simulink model "tx80211a2l"  (R2015b)
settings: Solver=FixedStepDiscrete  SolverMode=SingleTasking  StartTime=0.0  StopTime=46*tpf  RelTol=1e-3
PreLoadFcn:
  | [stx, stb, spi, spq, ntf, cii, cpp, css] = tx80211a_r0;
InitFcn:
  | if ~exist('srx','var')
  | [stx, stb, spi, spq, ntf, cii, cpp, css] = tx80211a_r0;
  | end
  | bitrate = 6e6; % 6 Mbits per second
  | crf = 2; % constant redundancy factor (from conv enc)
  | nepsc = 16; % #empty+pilot subcarriers
  | ncps = 16; % #cyclic prefix samples
  | ndbpf = 24; % #data bits per frame
  | ncbpf = ndbpf * crf; % #coded bits per frame
  | nscpf = ncbpf + nepsc; % #subcarriers per frame
  | nspf = nscpf + 16; % #samples per frame
  | tps = 1e-6; %tpf/nspf; % sample time
  | tpf = tps*nspf; %ndbpf/bitrate; % frame time
undefined symbols (not defined in the file): cpp, css, ntf, Radix, spi, spq, stb
libraries: hdlsllib x30, simulink x20, commdigbbndpm3 x1, commcnvcod2 x1, dspxfrm3 x1
settings Model: Creator=wchen  LastModifiedBy=bdroz
settings SolverCC: PositivePriorityOrder=on
settings DataIOCC: SaveFormat=Array  SaveOutput=off  SignalLogging=off  SaveTime=off
settings OptimizationCC: BlockReduction=off  ConditionallyExecuteInputs=off  DefaultParameterBehavior=Inlined  ExpressionDepthLimit=2147483647  OptimizeModelRefInitCode=on  LifeSpan=1  MaxStackSize=64
settings DebuggingCC: AlgebraicLoopMsg=error  UnderspecifiedInitializationDetection=Classic  MergeDetectMultiDrivingBlocksExec=none  SolverPrmCheckMsg=warning  SingleTaskRateTransMsg=error  ParameterPrecisionLossMsg=none  AllowSymbolicDim=on  StateNameClashWarn=warning
settings HardwareCC: ProdBitPerPointer=32  ProdLargestAtomicFloat=None  ProdIntDivRoundTo=Undefined  ProdEndianess=Unspecified  ProdWordSize=32  ProdHWDeviceType=ASIC/FPGA->ASIC/FPGA  TargetBitPerPointer=64  TargetLongLongMode=on  TargetIntDivRoundTo=Zero  TargetEndianess=LittleEndian  TargetWordSize=64  TargetHWDeviceType=MATLAB Host  ProdEqTarget=off
settings RTWCC: SystemTargetFile=ert.tlc  TemplateMakefile=ert_default_tmf  Description=Embedded Coder  GenerateReport=on  Toolchain=Xilinx Software Development Kit (SDK)  IncludeHyperlinkInReport=on  LaunchReport=on  GenerateTraceInfo=on  GenerateTraceReport=on  GenerateTraceReportSl=on  GenerateTraceReportSf=on  GenerateTraceReportEml=on
settings CodeAppCC: ForceParamTrailComments=on  IgnoreCustomStorageClasses=off  OperatorAnnotations=on  SimulinkDataObjDesc=on  SFDataObjDesc=on  MATLABFcnDesc=on  InsertBlockDesc=on  MATLABSourceComments=on
settings ERTTargetCC: ERTCustomFileTemplate=example_file_process.tlc  ConvertIfToSwitch=on  SuppressUnreachableDefaultCases=on
settings ConfigComp: CovModelRefEnable=Off

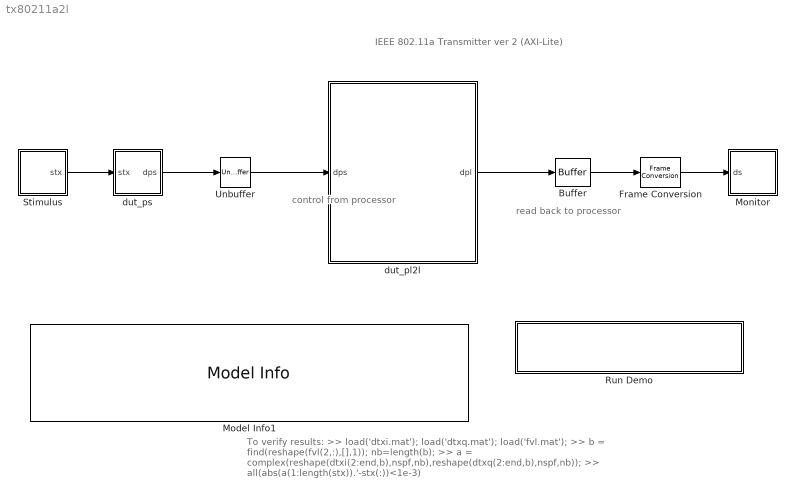
== system tx80211a2l ==
  note: control from
      | processor
  note: IEEE 802.11a Transmitter ver 2 (AXI-Lite)
  note: read back to
      | processor
  note: To verify results:
      | >> load('dtxi.mat'); load('dtxq.mat'); load('fvl.mat');
      | >> b = find(reshape(fvl(2,:),[],1)); nb=length(b);
      | >> a = complex(reshape(dtxi(2:end,b),nspf,nb),reshape(dtxq(2:end,b),nspf,nb));
      | >> all(abs(a(1:length(stx)).'-stx(:))<1e-3)
  Buffer : Buffer  N=80  TreatMby1Signals=One channel  OutputFrames=off
  Frame Conversion : FrameConversion  InheritSamplingMode=off  OutFrame=Sample-based
  Model Info1 : simulink/Model-Wide Utilities/Model Info  Frame=on  DisplayStringWithTags=|  HorizontalTextAlignment=Left  LeftAlignmentValue=0.02  SourceBlockDiagram=tx80211a2l  TagMaxNumber=20
      | This example shows how to use HDL Workflow Advisor to 
      | generate a custom IP core for Zynq SoC evaluation board.
      | 
      | In MATLAB, type the following:
      |   hdladvisor('tx80211a2l/dut_pl2l')
  Monitor : Subsystem
  Run Demo : Subsystem
      settings: OpenFcn=hdladvisor([bdroot, '/led_counter'])
      mask Display: disp('Launch HDL Workflow Advisor')
  Stimulus : Subsystem
  Unbuffer : Unbuffer  SampleBasedProcessing=Same as frame based
  dut_pl2l : Subsystem  TreatAsAtomicUnit=on
  dut_ps : Subsystem
  wires:
  Buffer/1 -> Frame Conversion/1
  dut_pl2l/1(dpl) -> Buffer/1
  Stimulus/1(stx) -> dut_ps/1(stx)
  dut_ps/1(dps) -> Unbuffer/1
  Unbuffer/1 -> dut_pl2l/1(dps)
  Frame Conversion/1 -> Monitor/1(ds)

== system tx80211a2l/Monitor ==
  ds : Inport
  Compare To Constant : simulink/Logic and Bit Operations/Compare To Constant  relop=>  const=uint16(0)  OutDataTypeStr=boolean
  Counter Free-Running : simulink/Sources/Counter Free-Running  NumBits=16  tsamp=tpf
  Unpack_int32_into_fix16c1b : Subsystem
  write_srb_to_file : Subsystem
  wires:
  Compare To Constant/1 -> write_srb_to_file/Enable
  Counter Free-Running/1 -> Compare To Constant/1
  ds/1 -> Unpack_int32_into_fix16c1b/1(di32)
  Unpack_int32_into_fix16c1b/2(fvd) -> write_srb_to_file/2(fvl)
  Unpack_int32_into_fix16c1b/1(dts) -> write_srb_to_file/1(srb)

== system tx80211a2l/Run Demo ==

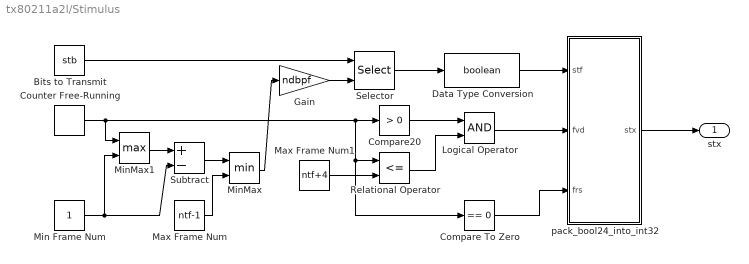
== system tx80211a2l/Stimulus ==
  Bits to Transmit : Constant  Value=stb  SampleTime=tpf
  Compare To Zero : simulink/Logic and Bit Operations/Compare To Zero  relop===  OutDataTypeStr=boolean
  Compare20 : simulink/Logic and Bit Operations/Compare To Zero  relop=>  OutDataTypeStr=boolean
  Counter Free-Running : simulink/Sources/Counter Free-Running  NumBits=16  tsamp=tpf
  Data Type Conversion : DataTypeConversion  OutDataTypeStr=boolean
  Gain : Gain  Gain=ndbpf  OutDataTypeStr=uint16
  Logical Operator : Logic  AllPortsSameDT=off  OutDataTypeStr=boolean
  Max Frame Num : Constant  Value=ntf-1  OutDataTypeStr=uint16  SampleTime=tpf
  Max Frame Num1 : Constant  Value=ntf+4  OutDataTypeStr=uint16  SampleTime=tpf
  Min Frame Num : Constant  OutDataTypeStr=uint16  SampleTime=tpf
  MinMax : MinMax  Inputs=2  OutDataTypeStr=uint16
  MinMax1 : MinMax  Function=max  Inputs=2
  Relational Operator : RelationalOperator  Operator=<=  OutDataTypeStr=boolean
  Selector : Selector  IndexMode=Zero-based  InputPortWidth=864  IndexOptions=Starting index (port)  Indices=[1 3]  OutputSizes=24
  Subtract : Sum  Inputs=+-  OutDataTypeStr=uint16
  pack_bool24_into_int32 : Subsystem
  stx : Outport
  wires:
  Compare To Zero/1 -> pack_bool24_into_int32/3(frs)
  MinMax1/1 -> Subtract/1
  Subtract/1 -> MinMax/1
  Min Frame Num/1 -> MinMax1/2, Subtract/2
  pack_bool24_into_int32/1(stx) -> stx/1
  Data Type Conversion/1 -> pack_bool24_into_int32/1(stf)
  Selector/1 -> Data Type Conversion/1
  Gain/1 -> Selector/2
  Bits to Transmit/1 -> Selector/1
  MinMax/1 -> Gain/1
  Max Frame Num/1 -> MinMax/2
  Counter Free-Running/1 -> Compare20/1, Relational Operator/1, Compare To Zero/1, MinMax1/1
  Compare20/1 -> Logical Operator/1
  Relational Operator/1 -> Logical Operator/2
  Logical Operator/1 -> pack_bool24_into_int32/2(fvd)
  Max Frame Num1/1 -> Relational Operator/2

== system tx80211a2l/dut_pl2l ==
  dps : Inport
  Preamble Switch : Subsystem  TreatAsAtomicUnit=on
  Unpack_int32_into_fix16c2b : Subsystem
  pack_fpt16c1b_into_int32 : Subsystem
  dpl : Outport
  wires:
  dps/1 -> Unpack_int32_into_fix16c2b/1(di32)
  Unpack_int32_into_fix16c2b/1(dts) -> Preamble Switch/1(s8s)
  Unpack_int32_into_fix16c2b/2(fvd) -> Preamble Switch/2(f8v)
  Preamble Switch/1(s9s) -> pack_fpt16c1b_into_int32/1(dtf16c)
  pack_fpt16c1b_into_int32/1(dti32) -> dpl/1
  Preamble Switch/2(f9v) -> pack_fpt16c1b_into_int32/2(fvd)
  Unpack_int32_into_fix16c2b/3(frs) -> Preamble Switch/3(frs)

== system tx80211a2l/dut_ps ==
  stx : Inport
  Logical AND : Logic  IconShape=distinctive  AllPortsSameDT=off  OutDataTypeStr=boolean
  pack_fpt16c_into_int32 : Subsystem
  prepare_frame_ps : Subsystem  TreatAsAtomicUnit=on
  unpack_int32_into_bool24 : Subsystem
  dps : Outport
  wires:
  stx/1 -> unpack_int32_into_bool24/1(di32)
  unpack_int32_into_bool24/3(frs) -> pack_fpt16c_into_int32/3(frs), prepare_frame_ps/2(frs)
  unpack_int32_into_bool24/1(stx) -> prepare_frame_ps/1(stb)
  unpack_int32_into_bool24/2(fvd) -> Logical AND/2, prepare_frame_ps/Enable
  prepare_frame_ps/2(fvo) -> Logical AND/1
  prepare_frame_ps/1(dts) -> pack_fpt16c_into_int32/1(dtf16c)
  Logical AND/1 -> pack_fpt16c_into_int32/2(fvd)
  pack_fpt16c_into_int32/1(dti32) -> dps/1

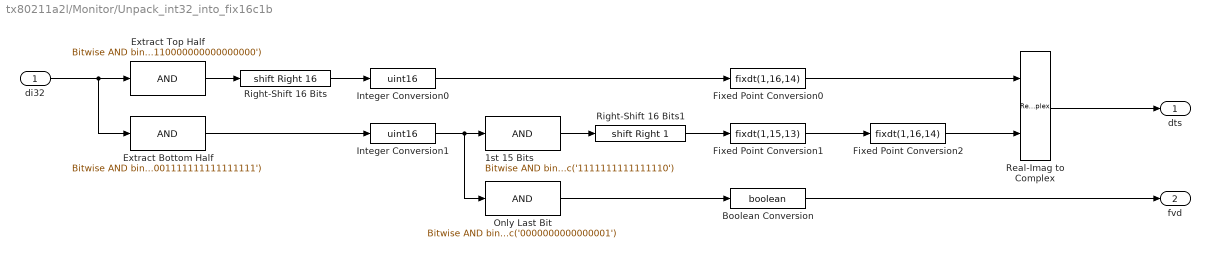
== system tx80211a2l/Monitor/Unpack_int32_into_fix16c1b ==
  di32 : Inport
  1st 15 Bits : simulink/Logic and Bit Operations/Bitwise Operator  logicop=AND  UseBitMask=on  BitMask=bin2dec('1111111111111110')  BitMaskRealWorld=Stored Integer
  Boolean Conversion : DataTypeConversion  OutDataTypeStr=boolean  ConvertRealWorld=Stored Integer (SI)
  Extract Bottom Half : simulink/Logic and Bit Operations/Bitwise Operator  logicop=AND  UseBitMask=on  BitMask=bin2dec('00000000000000001111111111111111')  BitMaskRealWorld=Stored Integer
  Extract Top Half : simulink/Logic and Bit Operations/Bitwise Operator  logicop=AND  UseBitMask=on  BitMask=bin2dec('11111111111111110000000000000000')  BitMaskRealWorld=Stored Integer
  Fixed Point Conversion0 : DataTypeConversion  OutDataTypeStr=fixdt(1,16,14)  ConvertRealWorld=Stored Integer (SI)
      settings: AttributesFormatString=%<OutDataTypeStr>
  Fixed Point Conversion1 : DataTypeConversion  OutDataTypeStr=fixdt(1,15,13)  ConvertRealWorld=Stored Integer (SI)
      settings: AttributesFormatString=%<OutDataTypeStr>
  Fixed Point Conversion2 : DataTypeConversion  OutDataTypeStr=fixdt(1,16,14)
      settings: AttributesFormatString=%<OutDataTypeStr>
  Integer Conversion0 : DataTypeConversion  OutDataTypeStr=uint16  ConvertRealWorld=Stored Integer (SI)
  Integer Conversion1 : DataTypeConversion  OutDataTypeStr=uint16  ConvertRealWorld=Stored Integer (SI)
  Only Last Bit : simulink/Logic and Bit Operations/Bitwise Operator  logicop=AND  UseBitMask=on  BitMask=bin2dec('0000000000000001')  BitMaskRealWorld=Stored Integer
  Real-Imag to Complex : RealImagToComplex
  Right-Shift 16 Bits : ArithShift  BitShiftNumber=16  BitShiftDirection=Right  DiagnosticForOORShift=Error
  Right-Shift 16 Bits1 : ArithShift  BitShiftNumber=1  BitShiftDirection=Right  DiagnosticForOORShift=Error
  dts : Outport
  fvd : Outport  Port=2
  wires:
  Real-Imag to Complex/1 -> dts/1
  Only Last Bit/1 -> Boolean Conversion/1
  Boolean Conversion/1 -> fvd/1
  Fixed Point Conversion0/1 -> Real-Imag to Complex/1
  Fixed Point Conversion2/1 -> Real-Imag to Complex/2
  Extract Bottom Half/1 -> Integer Conversion1/1
  di32/1 -> Extract Bottom Half/1, Extract Top Half/1
  1st 15 Bits/1 -> Right-Shift 16 Bits1/1
  Right-Shift 16 Bits/1 -> Integer Conversion0/1
  Extract Top Half/1 -> Right-Shift 16 Bits/1
  Integer Conversion1/1 -> 1st 15 Bits/1, Only Last Bit/1
  Integer Conversion0/1 -> Fixed Point Conversion0/1
  Fixed Point Conversion1/1 -> Fixed Point Conversion2/1
  Right-Shift 16 Bits1/1 -> Fixed Point Conversion1/1

== system tx80211a2l/Monitor/write_srb_to_file ==
  srb : Inport
  fvl : Inport  Port=2
  Enable : EnablePort
  Complex to Real-Imag : ComplexToRealImag
  Data Type Conversion : DataTypeConversion  OutDataTypeStr=double
  Data Type Conversion1 : DataTypeConversion  OutDataTypeStr=double
  To File : ToFile  Filename=dtxi.mat  MatrixName=dtxi  SampleTime=tpf
  To File1 : ToFile  Filename=fvl.mat  MatrixName=fvl  SampleTime=tpf
  To File2 : ToFile  Filename=dtxq.mat  MatrixName=dtxq  SampleTime=tpf
  wires:
  fvl/1 -> Data Type Conversion1/1
  Data Type Conversion1/1 -> To File1/1
  srb/1 -> Data Type Conversion/1
  Data Type Conversion/1 -> Complex to Real-Imag/1
  Complex to Real-Imag/1 -> To File/1
  Complex to Real-Imag/2 -> To File2/1

== system tx80211a2l/Stimulus/pack_bool24_into_int32 ==
  stf : Inport
  fvd : Inport  Port=2
  frs : Inport  Port=3
  Bit Concat : hdlsllib/HDL Operations/Bit Concat  numInputs=1
  Constant : Constant  Value=false(6,1)  OutDataTypeStr=boolean  SampleTime=tpf
  Vector Concatenate : Concatenate  NumInputs=4
  stx : Outport
  wires:
  Vector Concatenate/1 -> Bit Concat/1
  stf/1 -> Vector Concatenate/1
  fvd/1 -> Vector Concatenate/3
  frs/1 -> Vector Concatenate/4
  Constant/1 -> Vector Concatenate/2
  Bit Concat/1 -> stx/1

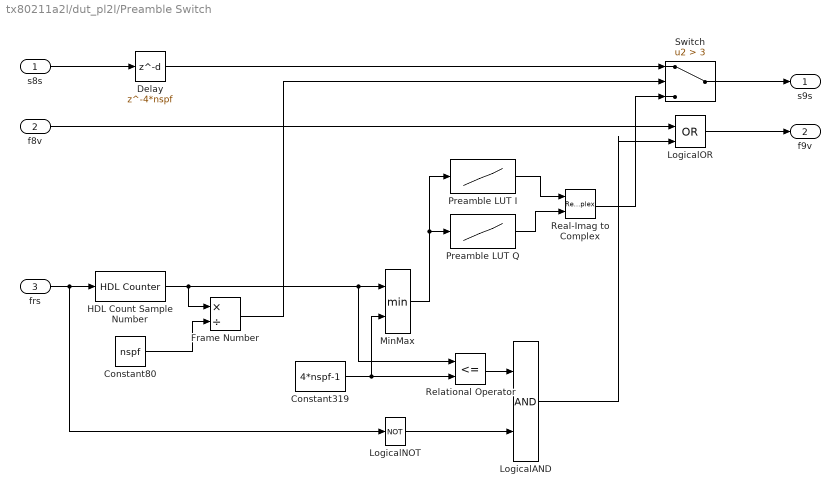
== system tx80211a2l/dut_pl2l/Preamble Switch ==
  s8s : Inport
  f8v : Inport  Port=2
  frs : Inport  Port=3
  Constant319 : Constant  Value=4*nspf-1  OutDataTypeStr=uint16  SampleTime=tps
  Constant80 : Constant  Value=nspf  OutDataTypeStr=uint8  SampleTime=tps
  Delay : Delay  DelayLength=4*nspf  SampleTime=tps
  Frame Number : Product  Inputs=*/  OutDataTypeStr=uint16  SaturateOnIntegerOverflow=on  RndMeth=Zero
  HDL Count Sample Number : hdlsllib/HDL Operations/HDL Counter  CountType=Free running  CountInit=0  CountStep=1  CountMax=3  CountFromType=Initial value  CountFrom=0  CountResetPort=on  CountLoadPort=off  CountEnbPort=off  CountDirPort=off  CountDataType=Unsigned  CountWordLen=16  CountFracLen=0  CountSampTime=1
  LogicalAND : Logic  IconShape=distinctive  AllPortsSameDT=off  OutDataTypeStr=boolean
  LogicalNOT : Logic  Operator=NOT  IconShape=distinctive  AllPortsSameDT=off  OutDataTypeStr=boolean
  LogicalOR : Logic  Operator=OR  IconShape=distinctive  AllPortsSameDT=off  OutDataTypeStr=boolean
  MinMax : MinMax  Inputs=2
  Preamble LUT I : Lookup_n-D  NumberOfTableDimensions=1  BreakpointsForDimension1=[0:1:319]  BreakpointsForDimension1FirstPoint=10  BreakpointsForDimension2FirstPoint=10  BreakpointsForDimension1Spacing=12  BreakpointsForDimension2Spacing=12  IndexSearchMethod=Evenly spaced points  Table=spi  InterpMethod=Flat  DiagnosticForOutOfRangeInput=Error  InternalRulePriority=Speed  OutDataTypeStr=fixdt(1,16,14)  RndMeth=Simplest  InputSameDT=on
  Preamble LUT Q : Lookup_n-D  NumberOfTableDimensions=1  BreakpointsForDimension1=[0:1:319]  BreakpointsForDimension1FirstPoint=10  BreakpointsForDimension2FirstPoint=10  BreakpointsForDimension1Spacing=12  BreakpointsForDimension2Spacing=12  IndexSearchMethod=Evenly spaced points  Table=spq  TableDataTypeStr=fixdt(1,16,14)  InterpMethod=Flat  DiagnosticForOutOfRangeInput=Error  InternalRulePriority=Speed  OutDataTypeStr=fixdt(1,16,14)  RndMeth=Simplest  InputSameDT=on
  Real-Imag to Complex : RealImagToComplex
  Relational Operator : RelationalOperator  Operator=<=  OutDataTypeStr=boolean
  Switch : Switch  Criteria=u2 > Threshold  Threshold=3
  s9s : Outport
  f9v : Outport  Port=2
  wires:
  frs/1 -> LogicalNOT/1, HDL Count Sample Number/1
  Switch/1 -> s9s/1
  s8s/1 -> Delay/1
  Real-Imag to Complex/1 -> Switch/3
  Constant80/1 -> Frame Number/2
  Delay/1 -> Switch/1
  Frame Number/1 -> Switch/2
  HDL Count Sample Number/1 -> Relational Operator/1, MinMax/1, Frame Number/1
  Constant319/1 -> MinMax/2, Relational Operator/2
  MinMax/1 -> Preamble LUT Q/1, Preamble LUT I/1
  LogicalOR/1 -> f9v/1
  LogicalNOT/1 -> LogicalAND/2
  Relational Operator/1 -> LogicalAND/1
  LogicalAND/1 -> LogicalOR/2
  f8v/1 -> LogicalOR/1
  Preamble LUT I/1 -> Real-Imag to Complex/1
  Preamble LUT Q/1 -> Real-Imag to Complex/2

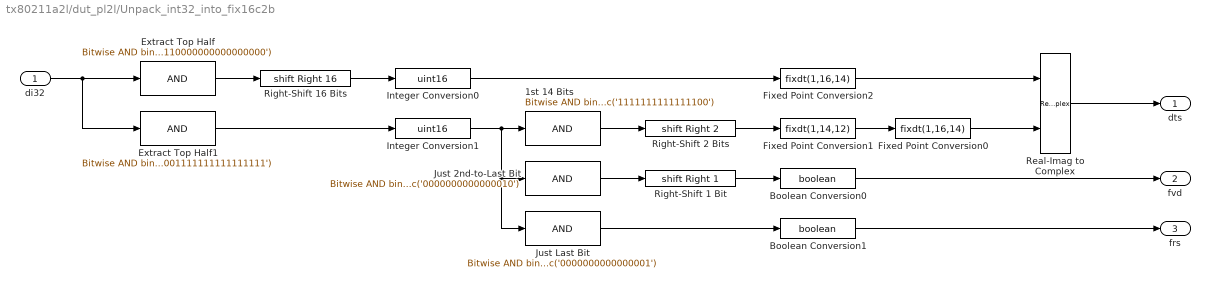
== system tx80211a2l/dut_pl2l/Unpack_int32_into_fix16c2b ==
  di32 : Inport
  1st 14 Bits : simulink/Logic and Bit Operations/Bitwise Operator  logicop=AND  UseBitMask=on  BitMask=bin2dec('1111111111111100')  BitMaskRealWorld=Stored Integer
  Boolean Conversion0 : DataTypeConversion  OutDataTypeStr=boolean  ConvertRealWorld=Stored Integer (SI)
  Boolean Conversion1 : DataTypeConversion  OutDataTypeStr=boolean  ConvertRealWorld=Stored Integer (SI)
  Extract Top Half : simulink/Logic and Bit Operations/Bitwise Operator  logicop=AND  UseBitMask=on  BitMask=bin2dec('11111111111111110000000000000000')  BitMaskRealWorld=Stored Integer
  Extract Top Half1 : simulink/Logic and Bit Operations/Bitwise Operator  logicop=AND  UseBitMask=on  BitMask=bin2dec('00000000000000001111111111111111')  BitMaskRealWorld=Stored Integer
  Fixed Point Conversion0 : DataTypeConversion  OutDataTypeStr=fixdt(1,16,14)  LockScale=on
      settings: AttributesFormatString=%<OutDataTypeStr>
  Fixed Point Conversion1 : DataTypeConversion  OutDataTypeStr=fixdt(1,14,12)  ConvertRealWorld=Stored Integer (SI)  LockScale=on
      settings: AttributesFormatString=%<OutDataTypeStr>
  Fixed Point Conversion2 : DataTypeConversion  OutDataTypeStr=fixdt(1,16,14)  ConvertRealWorld=Stored Integer (SI)
      settings: AttributesFormatString=%<OutDataTypeStr>
  Integer Conversion0 : DataTypeConversion  OutDataTypeStr=uint16  ConvertRealWorld=Stored Integer (SI)
  Integer Conversion1 : DataTypeConversion  OutDataTypeStr=uint16  ConvertRealWorld=Stored Integer (SI)
  Just 2nd-to-Last Bit : simulink/Logic and Bit Operations/Bitwise Operator  logicop=AND  UseBitMask=on  BitMask=bin2dec('0000000000000010')  BitMaskRealWorld=Stored Integer
  Just Last Bit : simulink/Logic and Bit Operations/Bitwise Operator  logicop=AND  UseBitMask=on  BitMask=bin2dec('0000000000000001')  BitMaskRealWorld=Stored Integer
  Real-Imag to Complex : RealImagToComplex
  Right-Shift 1 Bit : ArithShift  BitShiftNumber=1  BitShiftDirection=Right  DiagnosticForOORShift=Error
  Right-Shift 16 Bits : ArithShift  BitShiftNumber=16  BitShiftDirection=Right  DiagnosticForOORShift=Error
  Right-Shift 2 Bits : ArithShift  BitShiftNumber=2  BitShiftDirection=Right  DiagnosticForOORShift=Error
  dts : Outport
  fvd : Outport  Port=2
  frs : Outport  Port=3
  wires:
  Real-Imag to Complex/1 -> dts/1
  Just 2nd-to-Last Bit/1 -> Right-Shift 1 Bit/1
  Boolean Conversion0/1 -> fvd/1
  Extract Top Half1/1 -> Integer Conversion1/1
  Just Last Bit/1 -> Boolean Conversion1/1
  Boolean Conversion1/1 -> frs/1
  di32/1 -> Extract Top Half1/1, Extract Top Half/1
  Fixed Point Conversion2/1 -> Real-Imag to Complex/1
  Fixed Point Conversion1/1 -> Fixed Point Conversion0/1
  Extract Top Half/1 -> Right-Shift 16 Bits/1
  1st 14 Bits/1 -> Right-Shift 2 Bits/1
  Right-Shift 1 Bit/1 -> Boolean Conversion0/1
  Integer Conversion0/1 -> Fixed Point Conversion2/1
  Right-Shift 16 Bits/1 -> Integer Conversion0/1
  Integer Conversion1/1 -> Just Last Bit/1, Just 2nd-to-Last Bit/1, 1st 14 Bits/1
  Right-Shift 2 Bits/1 -> Fixed Point Conversion1/1
  Fixed Point Conversion0/1 -> Real-Imag to Complex/2

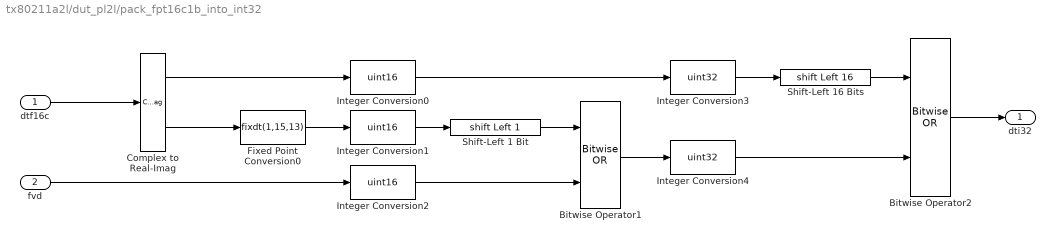
== system tx80211a2l/dut_pl2l/pack_fpt16c1b_into_int32 ==
  dtf16c : Inport
  fvd : Inport  Port=2
  Bitwise Operator1 : simulink/Logic and Bit Operations/Bitwise Operator  logicop=OR  UseBitMask=off  NumInputPorts=2  BitMask=bin2dec('11011001')  BitMaskRealWorld=Stored Integer
  Bitwise Operator2 : simulink/Logic and Bit Operations/Bitwise Operator  logicop=OR  UseBitMask=off  NumInputPorts=2  BitMask=bin2dec('11011001')  BitMaskRealWorld=Stored Integer
  Complex to Real-Imag : ComplexToRealImag
  Fixed Point Conversion0 : DataTypeConversion  OutDataTypeStr=fixdt(1,15,13)
      settings: AttributesFormatString=%<OutDataTypeStr>
  Integer Conversion0 : DataTypeConversion  OutDataTypeStr=uint16  ConvertRealWorld=Stored Integer (SI)
  Integer Conversion1 : DataTypeConversion  OutDataTypeStr=uint16  ConvertRealWorld=Stored Integer (SI)
  Integer Conversion2 : DataTypeConversion  OutDataTypeStr=uint16  ConvertRealWorld=Stored Integer (SI)
  Integer Conversion3 : DataTypeConversion  OutDataTypeStr=uint32  ConvertRealWorld=Stored Integer (SI)
  Integer Conversion4 : DataTypeConversion  OutDataTypeStr=uint32  ConvertRealWorld=Stored Integer (SI)
  Shift-Left 1 Bit : ArithShift  BitShiftNumber=1  BitShiftDirection=Left  DiagnosticForOORShift=Error
  Shift-Left 16 Bits : ArithShift  BitShiftNumber=16  BitShiftDirection=Left  DiagnosticForOORShift=Error
  dti32 : Outport
  wires:
  Bitwise Operator2/1 -> dti32/1
  dtf16c/1 -> Complex to Real-Imag/1
  Complex to Real-Imag/2 -> Fixed Point Conversion0/1
  fvd/1 -> Integer Conversion2/1
  Integer Conversion2/1 -> Bitwise Operator1/2
  Integer Conversion1/1 -> Shift-Left 1 Bit/1
  Bitwise Operator1/1 -> Integer Conversion4/1
  Complex to Real-Imag/1 -> Integer Conversion0/1
  Integer Conversion0/1 -> Integer Conversion3/1
  Integer Conversion3/1 -> Shift-Left 16 Bits/1
  Shift-Left 16 Bits/1 -> Bitwise Operator2/1
  Integer Conversion4/1 -> Bitwise Operator2/2
  Fixed Point Conversion0/1 -> Integer Conversion1/1
  Shift-Left 1 Bit/1 -> Bitwise Operator1/1

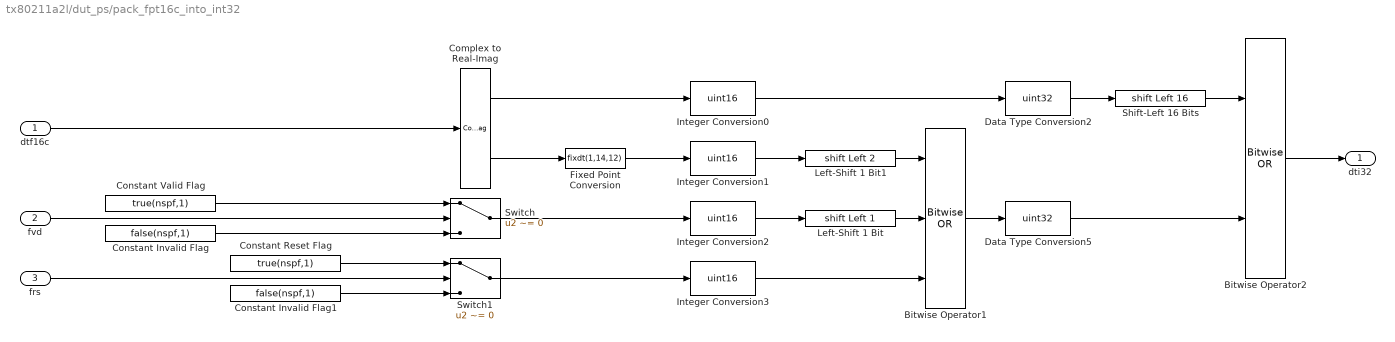
== system tx80211a2l/dut_ps/pack_fpt16c_into_int32 ==
  dtf16c : Inport
  fvd : Inport  Port=2
  frs : Inport  Port=3
  Bitwise Operator1 : simulink/Logic and Bit Operations/Bitwise Operator  logicop=OR  UseBitMask=off  NumInputPorts=3  BitMask=bin2dec('11011001')  BitMaskRealWorld=Stored Integer
  Bitwise Operator2 : simulink/Logic and Bit Operations/Bitwise Operator  logicop=OR  UseBitMask=off  NumInputPorts=2  BitMask=bin2dec('11011001')  BitMaskRealWorld=Stored Integer
  Complex to Real-Imag : ComplexToRealImag
  Constant Invalid Flag : Constant  Value=false(nspf,1)  OutDataTypeStr=boolean  SampleTime=tpf
  Constant Invalid Flag1 : Constant  Value=false(nspf,1)  OutDataTypeStr=boolean  SampleTime=tpf
  Constant Reset Flag : Constant  Value=true(nspf,1)  OutDataTypeStr=boolean  SampleTime=tpf
  Constant Valid Flag : Constant  Value=true(nspf,1)  OutDataTypeStr=boolean  SampleTime=tpf
  Data Type Conversion2 : DataTypeConversion  OutDataTypeStr=uint32  ConvertRealWorld=Stored Integer (SI)
  Data Type Conversion5 : DataTypeConversion  OutDataTypeStr=uint32  ConvertRealWorld=Stored Integer (SI)
  Fixed Point Conversion : DataTypeConversion  OutDataTypeStr=fixdt(1,14,12)
      settings: AttributesFormatString=%<OutDataTypeStr>
  Integer Conversion{0..3} (4 alike) : DataTypeConversion  OutDataTypeStr=uint16  ConvertRealWorld=Stored Integer (SI)
  Left-Shift 1 Bit : ArithShift  BitShiftNumber=1  BitShiftDirection=Left  DiagnosticForOORShift=Error
  Left-Shift 1 Bit1 : ArithShift  BitShiftNumber=2  BitShiftDirection=Left  DiagnosticForOORShift=Error
  Shift-Left 16 Bits : ArithShift  BitShiftNumber=16  BitShiftDirection=Left  DiagnosticForOORShift=Error
  Switch : Switch  Criteria=u2 ~= 0
  Switch1 : Switch  Criteria=u2 ~= 0
  dti32 : Outport
  wires:
  Bitwise Operator2/1 -> dti32/1
  Constant Valid Flag/1 -> Switch/1
  Constant Invalid Flag/1 -> Switch/3
  fvd/1 -> Switch/2
  Switch/1 -> Integer Conversion2/1
  dtf16c/1 -> Complex to Real-Imag/1
  Constant Reset Flag/1 -> Switch1/1
  Constant Invalid Flag1/1 -> Switch1/3
  frs/1 -> Switch1/2
  Switch1/1 -> Integer Conversion3/1
  Complex to Real-Imag/1 -> Integer Conversion0/1
  Complex to Real-Imag/2 -> Fixed Point Conversion/1
  Integer Conversion2/1 -> Left-Shift 1 Bit/1
  Integer Conversion1/1 -> Left-Shift 1 Bit1/1
  Left-Shift 1 Bit/1 -> Bitwise Operator1/2
  Integer Conversion3/1 -> Bitwise Operator1/3
  Bitwise Operator1/1 -> Data Type Conversion5/1
  Data Type Conversion2/1 -> Shift-Left 16 Bits/1
  Shift-Left 16 Bits/1 -> Bitwise Operator2/1
  Data Type Conversion5/1 -> Bitwise Operator2/2
  Integer Conversion0/1 -> Data Type Conversion2/1
  Fixed Point Conversion/1 -> Integer Conversion1/1
  Left-Shift 1 Bit1/1 -> Bitwise Operator1/1

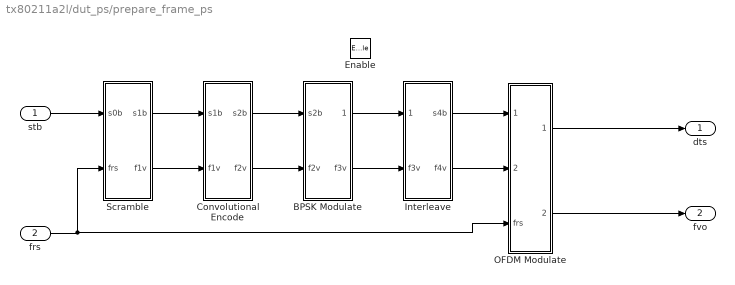
== system tx80211a2l/dut_ps/prepare_frame_ps ==
  stb : Inport
  frs : Inport  Port=2
  Enable : EnablePort
  BPSK Modulate : Subsystem  TreatAsAtomicUnit=on
  Convolutional Encode : Subsystem  TreatAsAtomicUnit=on
  Interleave : Subsystem  TreatAsAtomicUnit=on
  OFDM Modulate : Subsystem  TreatAsAtomicUnit=on
  Scramble : Subsystem  TreatAsAtomicUnit=on
  dts : Outport
  fvo : Outport  Port=2  InitialOutput=0
  wires:
  stb/1 -> Scramble/1(s0b)
  frs/1 -> OFDM Modulate/3(frs), Scramble/2(frs)
  Scramble/1(s1b) -> Convolutional Encode/1(s1b)
  Scramble/2(f1v) -> Convolutional Encode/2(f1v)
  Convolutional Encode/1(s2b) -> BPSK Modulate/1(s2b)
  Convolutional Encode/2(f2v) -> BPSK Modulate/2(f2v)
  BPSK Modulate/1(s3m) -> Interleave/1(s3m)
  BPSK Modulate/2(f3v) -> Interleave/2(f3v)
  Interleave/1(s4b) -> OFDM Modulate/1(s4m)
  Interleave/2(f4v) -> OFDM Modulate/2(f4v)
  OFDM Modulate/2(f8v) -> fvo/1
  OFDM Modulate/1(s8s) -> dts/1

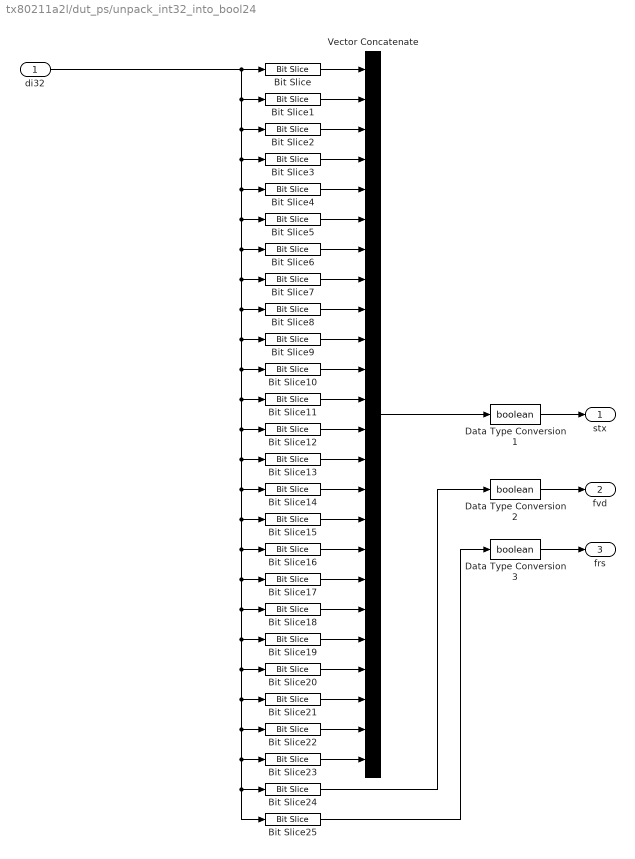
== system tx80211a2l/dut_ps/unpack_int32_into_bool24 ==
  di32 : Inport
  Bit Slice : hdlsllib/HDL Operations/Bit Slice  lidx=31  ridx=31
      settings: AttributesFormatString=%<lidx>
  Bit Slice1 : hdlsllib/HDL Operations/Bit Slice  lidx=30  ridx=30
      settings: AttributesFormatString=%<lidx>
  Bit Slice10 : hdlsllib/HDL Operations/Bit Slice  lidx=21  ridx=21
      settings: AttributesFormatString=%<lidx>
  Bit Slice11 : hdlsllib/HDL Operations/Bit Slice  lidx=20  ridx=20
      settings: AttributesFormatString=%<lidx>
  Bit Slice12 : hdlsllib/HDL Operations/Bit Slice  lidx=19  ridx=19
      settings: AttributesFormatString=%<lidx>
  Bit Slice13 : hdlsllib/HDL Operations/Bit Slice  lidx=18  ridx=18
      settings: AttributesFormatString=%<lidx>
  Bit Slice14 : hdlsllib/HDL Operations/Bit Slice  lidx=17  ridx=17
      settings: AttributesFormatString=%<lidx>
  Bit Slice15 : hdlsllib/HDL Operations/Bit Slice  lidx=16  ridx=16
      settings: AttributesFormatString=%<lidx>
  Bit Slice16 : hdlsllib/HDL Operations/Bit Slice  lidx=15  ridx=15
      settings: AttributesFormatString=%<lidx>
  Bit Slice17 : hdlsllib/HDL Operations/Bit Slice  lidx=14  ridx=14
      settings: AttributesFormatString=%<lidx>
  Bit Slice18 : hdlsllib/HDL Operations/Bit Slice  lidx=13  ridx=13
      settings: AttributesFormatString=%<lidx>
  Bit Slice19 : hdlsllib/HDL Operations/Bit Slice  lidx=12  ridx=12
      settings: AttributesFormatString=%<lidx>
  Bit Slice2 : hdlsllib/HDL Operations/Bit Slice  lidx=29  ridx=29
      settings: AttributesFormatString=%<lidx>
  Bit Slice20 : hdlsllib/HDL Operations/Bit Slice  lidx=11  ridx=11
      settings: AttributesFormatString=%<lidx>
  Bit Slice21 : hdlsllib/HDL Operations/Bit Slice  lidx=10  ridx=10
      settings: AttributesFormatString=%<lidx>
  Bit Slice22 : hdlsllib/HDL Operations/Bit Slice  lidx=9  ridx=9
      settings: AttributesFormatString=%<lidx>
  Bit Slice23 : hdlsllib/HDL Operations/Bit Slice  lidx=8  ridx=8
      settings: AttributesFormatString=%<lidx>
  Bit Slice24 : hdlsllib/HDL Operations/Bit Slice  lidx=1  ridx=1
      settings: AttributesFormatString=%<lidx>
  Bit Slice25 : hdlsllib/HDL Operations/Bit Slice  lidx=0  ridx=0
      settings: AttributesFormatString=%<lidx>
  Bit Slice3 : hdlsllib/HDL Operations/Bit Slice  lidx=28  ridx=28
      settings: AttributesFormatString=%<lidx>
  Bit Slice4 : hdlsllib/HDL Operations/Bit Slice  lidx=27  ridx=27
      settings: AttributesFormatString=%<lidx>
  Bit Slice5 : hdlsllib/HDL Operations/Bit Slice  lidx=26  ridx=26
      settings: AttributesFormatString=%<lidx>
  Bit Slice6 : hdlsllib/HDL Operations/Bit Slice  lidx=25  ridx=25
      settings: AttributesFormatString=%<lidx>
  Bit Slice7 : hdlsllib/HDL Operations/Bit Slice  lidx=24  ridx=24
      settings: AttributesFormatString=%<lidx>
  Bit Slice8 : hdlsllib/HDL Operations/Bit Slice  lidx=23  ridx=23
      settings: AttributesFormatString=%<lidx>
  Bit Slice9 : hdlsllib/HDL Operations/Bit Slice  lidx=22  ridx=22
      settings: AttributesFormatString=%<lidx>
  Data Type Conversion1 : DataTypeConversion  OutDataTypeStr=boolean
  Data Type Conversion2 : DataTypeConversion  OutDataTypeStr=boolean
  Data Type Conversion3 : DataTypeConversion  OutDataTypeStr=boolean
  Vector Concatenate : Concatenate  NumInputs=24
  stx : Outport
  fvd : Outport  Port=2
  frs : Outport  Port=3
  wires:
  Vector Concatenate/1 -> Data Type Conversion1/1
  Bit Slice25/1 -> Data Type Conversion3/1
  Bit Slice24/1 -> Data Type Conversion2/1
  di32/1 -> Bit Slice1/1, Bit Slice2/1, Bit Slice3/1, Bit Slice4/1, Bit Slice5/1, Bit Slice7/1, Bit Slice8/1, Bit Slice9/1, Bit Slice11/1, Bit Slice12/1, Bit Slice13/1, Bit Slice15/1, Bit Slice17/1, Bit Slice18/1, Bit Slice19/1, Bit Slice20/1, Bit Slice21/1, Bit Slice25/1, Bit Slice24/1, Bit Slice23/1, Bit Slice22/1, Bit Slice16/1, Bit Slice14/1, Bit Slice10/1, Bit Slice6/1, Bit Slice/1
  Bit Slice23/1 -> Vector Concatenate/24
  Bit Slice22/1 -> Vector Concatenate/23
  Bit Slice21/1 -> Vector Concatenate/22
  Bit Slice20/1 -> Vector Concatenate/21
  Bit Slice19/1 -> Vector Concatenate/20
  Bit Slice18/1 -> Vector Concatenate/19
  Bit Slice17/1 -> Vector Concatenate/18
  Bit Slice16/1 -> Vector Concatenate/17
  Bit Slice15/1 -> Vector Concatenate/16
  Bit Slice14/1 -> Vector Concatenate/15
  Bit Slice13/1 -> Vector Concatenate/14
  Bit Slice12/1 -> Vector Concatenate/13
  Bit Slice11/1 -> Vector Concatenate/12
  Bit Slice10/1 -> Vector Concatenate/11
  Bit Slice9/1 -> Vector Concatenate/10
  Bit Slice8/1 -> Vector Concatenate/9
  Bit Slice7/1 -> Vector Concatenate/8
  Bit Slice6/1 -> Vector Concatenate/7
  Bit Slice5/1 -> Vector Concatenate/6
  Bit Slice4/1 -> Vector Concatenate/5
  Bit Slice3/1 -> Vector Concatenate/4
  Bit Slice2/1 -> Vector Concatenate/3
  Bit Slice1/1 -> Vector Concatenate/2
  Bit Slice/1 -> Vector Concatenate/1
  Data Type Conversion1/1 -> stx/1
  Data Type Conversion2/1 -> fvd/1
  Data Type Conversion3/1 -> frs/1

== system tx80211a2l/dut_ps/prepare_frame_ps/BPSK Modulate ==
  s2b : Inport
  f2v : Inport  Port=2
  BPSK Modulator Baseband : commdigbbndpm3/BPSK Modulator Baseband  Ph=0  outDtype=Fixed-point  outWordLen=16  outUDDataType=sfix(16)  outFracLenMode=User-defined  outFracLen=14
  Logical NOT : Logic  Operator=NOT  IconShape=distinctive  AllPortsSameDT=off  OutDataTypeStr=boolean
  s3m : Outport
  f3v : Outport  Port=2
  wires:
  s2b/1 -> Logical NOT/1
  f2v/1 -> f3v/1
  Logical NOT/1 -> BPSK Modulator Baseband/1
  BPSK Modulator Baseband/1 -> s3m/1

== system tx80211a2l/dut_ps/prepare_frame_ps/Convolutional Encode ==
  s1b : Inport
  f1v : Inport  Port=2
  Convolutional Encoder : commcnvcod2/Convolutional Encoder  trellis=poly2trellis(7, [133,171])  opMode=Continuous  DelayedResetAction=on  hasIniStPort=off  hasFinStPort=off  usePuncVector=off  punctureVector=[1; 1; 0; 1; 0; 1]  reset=Unused parameter value
  s2b : Outport
  f2v : Outport  Port=2
  wires:
  f1v/1 -> f2v/1
  s1b/1 -> Convolutional Encoder/1
  Convolutional Encoder/1 -> s2b/1

== system tx80211a2l/dut_ps/prepare_frame_ps/Interleave ==
  s3m : Inport
  f3v : Inport  Port=2
  Selector : Selector  IndexMode=Zero-based  InputPortWidth=48  IndexOptions=Index vector (dialog)  Indices=cii  OutputSizes=1
  s4b : Outport
  f4v : Outport  Port=2
  wires:
  f3v/1 -> f4v/1
  s3m/1 -> Selector/1
  Selector/1 -> s4b/1

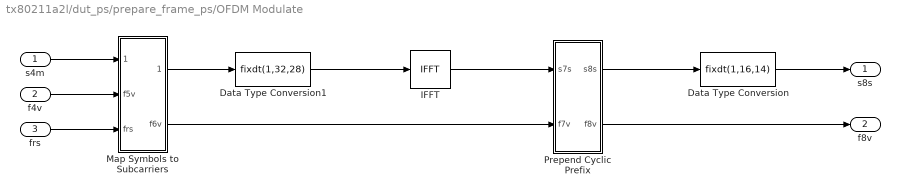
== system tx80211a2l/dut_ps/prepare_frame_ps/OFDM Modulate ==
  s4m : Inport
  f4v : Inport  Port=2
  frs : Inport  Port=3
  Data Type Conversion : DataTypeConversion  OutDataTypeStr=fixdt(1,16,14)  SaturateOnIntegerOverflow=on
  Data Type Conversion1 : DataTypeConversion  OutDataTypeStr=fixdt(1,32,28)  SaturateOnIntegerOverflow=on
  IFFT : dspxfrm3/IFFT  FFTImplementation=Radix-2  CompMethod=Table lookup  TableOpt=NEW  TableOptActive=Speed  BitRevOrder=off  cs_in=off  Normalize=on  InheritFFTLength=off  FFTLength=64  WrapInput=off  mode=Complex  outSamplingMode=Sample based  roundingMode=Round  overflowMode=on  firstCoeffMode=Specify word length  firstCoeffWordLength=32  firstCoeffFracLength=15  firstCoeffDataTypeStr=fixdt(1,32)  firstCoeffLastDataTypeStr=fixdt(1,32)  prodOutputMode=Binary point scaling  prodOutputWordLength=32  prodOutputFracLength=28  prodOutputDataTypeStr=fixdt(1,32,28)  prodOutputLastDataTypeStr=fixdt(1,32,28)  accumMode=Binary point scaling  accumWordLength=32  accumFracLength=28  accumDataTypeStr=fixdt(1,32,28)  accumLastDataTypeStr=fixdt(1,32,28)  outputMode=Binary point scaling  outputWordLength=32  outputFracLength=28  outputDataTypeStr=fixdt(1,32,28)  outputMin=[]  outputMax=[]  outputLastDataTypeStr=fixdt(1,32,28)
      settings: AttributesFormatString=%<FFTImplementation>, length %<FFTLength>  LockScale=on
  Map Symbols to Subcarriers : Subsystem  TreatAsAtomicUnit=on
  Prepend Cyclic Prefix : Subsystem  TreatAsAtomicUnit=on
  s8s : Outport
  f8v : Outport  Port=2
  wires:
  Prepend Cyclic Prefix/1(s8s) -> Data Type Conversion/1
  s4m/1 -> Map Symbols to Subcarriers/1(s5m)
  f4v/1 -> Map Symbols to Subcarriers/2(f5v)
  Prepend Cyclic Prefix/2(f8v) -> f8v/1
  frs/1 -> Map Symbols to Subcarriers/3(frs)
  Map Symbols to Subcarriers/2(f6v) -> Prepend Cyclic Prefix/2(f7v)
  Map Symbols to Subcarriers/1(s6m) -> Data Type Conversion1/1
  IFFT/1 -> Prepend Cyclic Prefix/1(s7s)
  Data Type Conversion1/1 -> IFFT/1
  Data Type Conversion/1 -> s8s/1

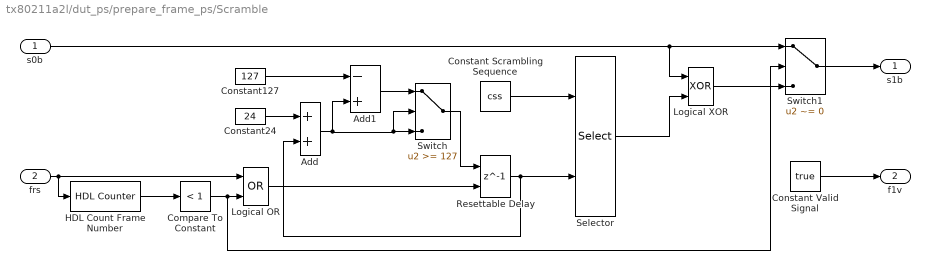
== system tx80211a2l/dut_ps/prepare_frame_ps/Scramble ==
  s0b : Inport
  frs : Inport  Port=2
  Add : Sum  AccumDataTypeStr=int16  OutDataTypeStr=int16  SaturateOnIntegerOverflow=on
  Add1 : Sum  Inputs=-+  AccumDataTypeStr=int16  OutDataTypeStr=int16  SaturateOnIntegerOverflow=on  LockScale=on
  Compare To Constant : simulink/Logic and Bit Operations/Compare To Constant  relop=<  const=1  OutDataTypeStr=boolean
  Constant Scrambling Sequence : Constant  Value=css  OutDataTypeStr=boolean  SampleTime=tpf
  Constant Valid Signal : Constant  Value=true  OutDataTypeStr=boolean  SampleTime=tpf
  Constant127 : Constant  Value=127  OutDataTypeStr=int16  SampleTime=tpf
  Constant24 : Constant  Value=24  OutDataTypeStr=int16  SampleTime=tpf
  HDL Count Frame Number : hdlsllib/HDL Operations/HDL Counter  CountType=Free running  CountInit=0  CountStep=1  CountMax=25  CountFromType=Initial value  CountFrom=0  CountResetPort=on  CountLoadPort=off  CountEnbPort=off  CountDirPort=off  CountDataType=Unsigned  CountWordLen=16  CountFracLen=0  CountSampTime=1
  Logical OR : Logic  Operator=OR  IconShape=distinctive  AllPortsSameDT=off  OutDataTypeStr=boolean
  Logical XOR : Logic  Operator=XOR  IconShape=distinctive  AllPortsSameDT=off  OutDataTypeStr=boolean
  Resettable Delay : Delay  DelayLength=1  InitialCondition=int16(0)  ExternalReset=Level  SampleTime=tpf
      settings: InputPortMap=u0,r5
  Selector : Selector  IndexMode=Zero-based  InputPortWidth=254  IndexOptions=Starting index (port)  Indices=[1 3]  OutputSizes=24
  Switch : Switch  Threshold=127
  Switch1 : Switch  Criteria=u2 ~= 0
  s1b : Outport
  f1v : Outport  Port=2
  wires:
  s0b/1 -> Switch1/1, Logical XOR/1
  frs/1 -> HDL Count Frame Number/1, Logical OR/1
  HDL Count Frame Number/1 -> Compare To Constant/1
  Compare To Constant/1 -> Switch1/2, Logical OR/2
  Resettable Delay/1 -> Add/2, Selector/2
  Constant Scrambling Sequence/1 -> Selector/1
  Selector/1 -> Logical XOR/2
  Constant Valid Signal/1 -> f1v/1
  Constant24/1 -> Add/1
  Switch/1 -> Resettable Delay/1
  Add/1 -> Add1/2, Switch/2, Switch/3
  Add1/1 -> Switch/1
  Constant127/1 -> Add1/1
  Logical OR/1 -> Resettable Delay/2
  Logical XOR/1 -> Switch1/3
  Switch1/1 -> s1b/1

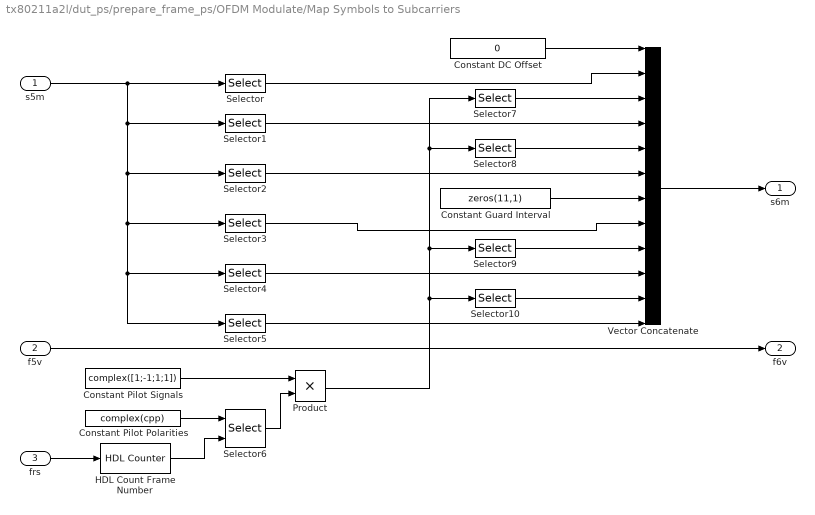
== system tx80211a2l/dut_ps/prepare_frame_ps/OFDM Modulate/Map Symbols to Subcarriers ==
  s5m : Inport
  f5v : Inport  Port=2
  frs : Inport  Port=3
  Constant DC Offset : Constant  Value=0  OutDataTypeStr=fixdt(1,16,14)  SampleTime=tpf
  Constant Guard Interval : Constant  Value=zeros(11,1)  OutDataTypeStr=fixdt(1,16,14)  SampleTime=tpf
  Constant Pilot Polarities : Constant  Value=complex(cpp)  OutDataTypeStr=fixdt(1,16,14)  SampleTime=tpf
  Constant Pilot Signals : Constant  Value=complex([1;-1;1;1])  OutDataTypeStr=fixdt(1,16,14)  SampleTime=tpf
  HDL Count Frame Number : hdlsllib/HDL Operations/HDL Counter  CountType=Free running  CountInit=0  CountStep=1  CountMax=25  CountFromType=Initial value  CountFrom=0  CountResetPort=on  CountLoadPort=off  CountEnbPort=off  CountDirPort=off  CountDataType=Unsigned  CountWordLen=8  CountFracLen=0  CountSampTime=1
  Product : Product  OutDataTypeStr=fixdt(1,16,14)
  Selector : Selector  IndexMode=Zero-based  InputPortWidth=48  IndexOptions=Index vector (dialog)  Indices=24:29  OutputSizes=1
  Selector1 : Selector  IndexMode=Zero-based  InputPortWidth=48  IndexOptions=Index vector (dialog)  Indices=30:42  OutputSizes=1
  Selector10 : Selector  IndexMode=Zero-based  InputPortWidth=4  IndexOptions=Index vector (dialog)  Indices=3  OutputSizes=1
  Selector2 : Selector  IndexMode=Zero-based  InputPortWidth=48  IndexOptions=Index vector (dialog)  Indices=43:47  OutputSizes=1
  Selector3 : Selector  IndexMode=Zero-based  InputPortWidth=48  IndexOptions=Index vector (dialog)  Indices=0:4  OutputSizes=1
  Selector4 : Selector  IndexMode=Zero-based  InputPortWidth=48  IndexOptions=Index vector (dialog)  Indices=5:17  OutputSizes=1
  Selector5 : Selector  IndexMode=Zero-based  InputPortWidth=48  IndexOptions=Index vector (dialog)  Indices=18:23  OutputSizes=1
  Selector6 : Selector  IndexMode=Zero-based  InputPortWidth=127  IndexOptions=Starting index (port)  Indices=[1 3]  OutputSizes=1
  Selector7 : Selector  IndexMode=Zero-based  InputPortWidth=4  IndexOptions=Index vector (dialog)  Indices=0  OutputSizes=1
  Selector8 : Selector  IndexMode=Zero-based  InputPortWidth=4  IndexOptions=Index vector (dialog)  Indices=1  OutputSizes=1
  Selector9 : Selector  IndexMode=Zero-based  InputPortWidth=4  IndexOptions=Index vector (dialog)  Indices=2  OutputSizes=1
  Vector Concatenate : Concatenate  NumInputs=12
  s6m : Outport
  f6v : Outport  Port=2
  wires:
  f5v/1 -> f6v/1
  s5m/1 -> Selector2/1, Selector3/1, Selector4/1, Selector5/1, Selector1/1, Selector/1
  frs/1 -> HDL Count Frame Number/1
  HDL Count Frame Number/1 -> Selector6/2
  Constant Pilot Polarities/1 -> Selector6/1
  Constant Pilot Signals/1 -> Product/1
  Selector6/1 -> Product/2
  Selector/1 -> Vector Concatenate/2
  Selector1/1 -> Vector Concatenate/4
  Selector2/1 -> Vector Concatenate/6
  Selector3/1 -> Vector Concatenate/8
  Selector4/1 -> Vector Concatenate/10
  Selector5/1 -> Vector Concatenate/12
  Constant DC Offset/1 -> Vector Concatenate/1
  Selector10/1 -> Vector Concatenate/11
  Selector9/1 -> Vector Concatenate/9
  Selector8/1 -> Vector Concatenate/5
  Selector7/1 -> Vector Concatenate/3
  Constant Guard Interval/1 -> Vector Concatenate/7
  Vector Concatenate/1 -> s6m/1
  Product/1 -> Selector10/1, Selector9/1, Selector8/1, Selector7/1

== system tx80211a2l/dut_ps/prepare_frame_ps/OFDM Modulate/Prepend Cyclic Prefix ==
  s7s : Inport
  f7v : Inport  Port=2
  Selector : Selector  IndexMode=Zero-based  InputPortWidth=64  IndexOptions=Index vector (dialog)  Indices=48:63  OutputSizes=1
  Vector Concatenate : Concatenate
  s8s : Outport
  f8v : Outport  Port=2
  wires:
  s7s/1 -> Vector Concatenate/2, Selector/1
  f7v/1 -> f8v/1
  Selector/1 -> Vector Concatenate/1
  Vector Concatenate/1 -> s8s/1
